simulink model "magnetorquer"  (R2022b)
settings: Solver=VariableStepAuto  StartTime=0.0  StopTime=10.0  RelTol=1e-3
libraries: matrix_library x1
settings Model: Creator=dell  LastModifiedBy=dell

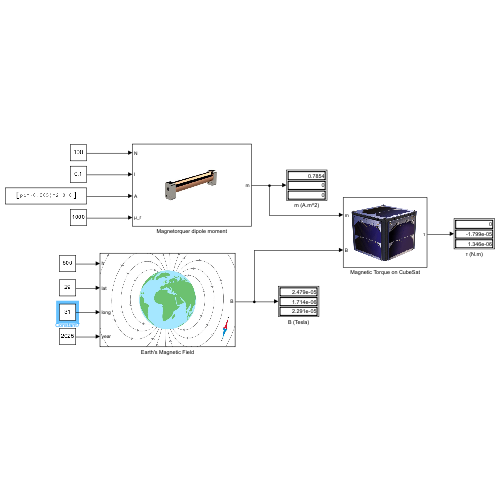
[thumbnail: Simulink's stored preview of the top-level diagram]
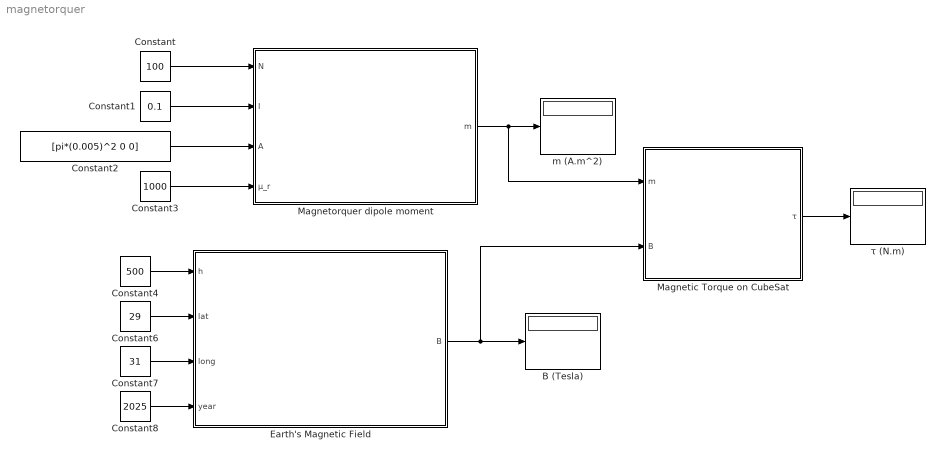
== system magnetorquer ==
  B (Tesla) : Display
  Constant : Constant  Value=100
  Constant1 : Constant  Value=0.1
  Constant2 : Constant  Value=[pi*(0.005)^2 0 0]
  Constant3 : Constant  Value=1000
  Constant4 : Constant  Value=500
  Constant6 : Constant  Value=29
  Constant7 : Constant  Value=31
  Constant8 : Constant  Value=2025
  Earth's Magnetic Field : Subsystem
      mask Display: image('$imagefile'); % Use "Edit Image" on toolstrip to change.
  Magnetic Torque on CubeSat : Subsystem
      mask Display: image('$imagefile'); % Use "Edit Image" on toolstrip to change.
  Magnetorquer dipole moment : Subsystem
      mask Display: image('$imagefile'); % Use "Edit Image" on toolstrip to change.
  m (A.m^2) : Display
  τ (N.m) : Display
  wires:
  Constant/1 -> Magnetorquer dipole moment/1(N)
  Constant1/1 -> Magnetorquer dipole moment/2(I)
  Constant2/1 -> Magnetorquer dipole moment/3(A)
  Constant3/1 -> Magnetorquer dipole moment/4(μ_r)
  Magnetorquer dipole moment/1(m) -> m (A.m^2)/1, Magnetic Torque on CubeSat/1(m)
  Earth's Magnetic Field/1(B) -> B (Tesla)/1, Magnetic Torque on CubeSat/2(B)
  Magnetic Torque on CubeSat/1(τ) -> τ (N.m)/1
  Constant4/1 -> Earth's Magnetic Field/1(h)
  Constant6/1 -> Earth's Magnetic Field/2(lat)
  Constant7/1 -> Earth's Magnetic Field/3(long)
  Constant8/1 -> Earth's Magnetic Field/4(year)

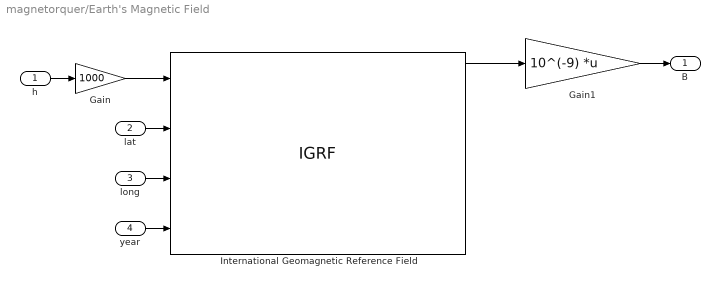
== system magnetorquer/Earth's Magnetic Field ==
  h : Inport
  lat : Inport  Port=2
  long : Inport  Port=3
  year : Inport  Port=4
  Gain : Gain  Gain=1000
  Gain1 : Gain  Gain=10^(-9)  Multiplication=Matrix(K*u)
  International Geomagnetic Reference Field : IGRF  month=January  day=1  year=2020
      settings: AttributesFormatString=%<generation>
  B : Outport
  wires:
  Gain/1 -> International Geomagnetic Reference Field/1
  h/1 -> Gain/1
  year/1 -> International Geomagnetic Reference Field/4
  long/1 -> International Geomagnetic Reference Field/3
  lat/1 -> International Geomagnetic Reference Field/2
  International Geomagnetic Reference Field/1 -> Gain1/1
  Gain1/1 -> B/1

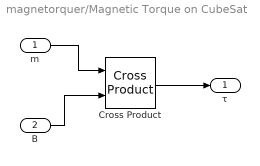
== system magnetorquer/Magnetic Torque on CubeSat ==
  m : Inport
  B : Inport  Port=2
  Cross Product : matrix_library/Cross Product
  τ : Outport
  wires:
  m/1 -> Cross Product/1
  B/1 -> Cross Product/2
  Cross Product/1 -> τ/1

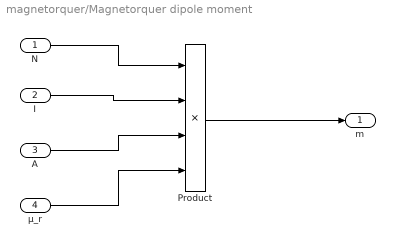
== system magnetorquer/Magnetorquer dipole moment ==
  N : Inport
  I : Inport  Port=2
  A : Inport  Port=3
  μ_r : Inport  Port=4
  Product : Product  Inputs=4
  m : Outport
  wires:
  N/1 -> Product/1
  I/1 -> Product/2
  A/1 -> Product/3
  μ_r/1 -> Product/4
  Product/1 -> m/1
